simulink model "ejemplo_af"  (R2018a)
settings: Solver=VariableStepAuto  StartTime=0.0  StopTime=100  MaxStep=1e-2  RelTol=1e-3
settings Model: Creator=carma  LastModifiedBy=carma

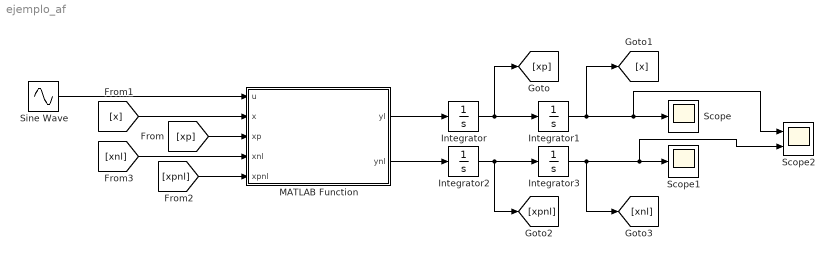
== system ejemplo_af ==
  Integrator{,1..3} (4 alike) : Integrator
  MATLAB Function : MATLAB Function  TreatAsAtomicUnit=on
  Scope : Scope
  Scope1 : Scope
  Scope2 : Scope  NumInputPorts=2
  Sine Wave : Sin  Amplitude=4  Frequency=0.1  SampleTime=0
  wires:
  Sine Wave/1 -> MATLAB Function/1(u)
  MATLAB Function/1(yl) -> Integrator/1
  Integrator/1 -> [xp], Integrator1/1
  Integrator1/1 -> [x], Scope2/1, Scope/1
  Integrator2/1 -> [xpnl], Integrator3/1
  MATLAB Function/2(ynl) -> Integrator2/1
  [xp] -> MATLAB Function/3(xp)
  [x] -> MATLAB Function/2(x)
  [xpnl] -> MATLAB Function/5(xpnl)
  [xnl] -> MATLAB Function/4(xnl)
  Integrator3/1 -> [xnl], Scope2/2, Scope1/1

== matlab function ejemplo_af/MATLAB Function ==
  data: u input; yl output; x input; xp input; xnl input; xpnl input; ynl output
function [yl,ynl]= fcn(u,x,xp,xnl,xpnl)
%parametros
m=10;
b=2;
k=5;
kp=100*k
yl=(u-k*x-b*xp)/m;
ynl=(u-k*(xnl+kp*xnl^3)-b*xpnl)/m;
